simulink model "Ackerman_simulation"  (R2024b)
settings: Solver=VariableStepAuto  StartTime=0.0  StopTime=inf  RelTol=1e-3
values from neighbouring files (symbols this model uses):
  psi_o = 0    [PursuitWaypoints.m]
  Ts = 200    [PursuitWaypoints.m]    (also in retardo.m = 0.01)
  X_end = refPose(end,1)    [PursuitWaypoints.m]
  X_o = refPose(1,1)    [PursuitWaypoints.m]
  xRef = interp1(1:length(xRef), xRef, puntos_finos, 'spline')'    [PursuitWaypoints.m]
  Y_end = -refPose(end,2)    [PursuitWaypoints.m]
  Y_o = -refPose(1,2)    [PursuitWaypoints.m]
  yRef = interp1(1:length(yRef), yRef, puntos_finos, 'spline')'    [PursuitWaypoints.m]
undefined symbols (not defined in the file or in its folder): DiscIntNeverNeededParam
libraries: simulink x6, robotalgslib x2, robotmobilelib x1
settings Model: Creator=johan  LastModifiedBy=johan
settings OptimizationCC: DefaultParameterBehavior=Inlined  GainParamInheritBuiltInType=on  UseFloatMulNetSlope=on  InlineInvariantSignals=on  EfficientFloat2IntCast=on
settings RTWCC: RTWVerbose=off  BuildConfiguration=Faster Runs
settings GRTTargetCC: MatFileLogging=off

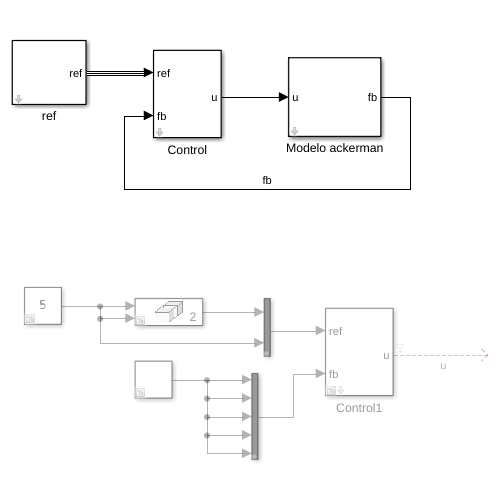
[thumbnail: Simulink's stored preview of the top-level diagram]
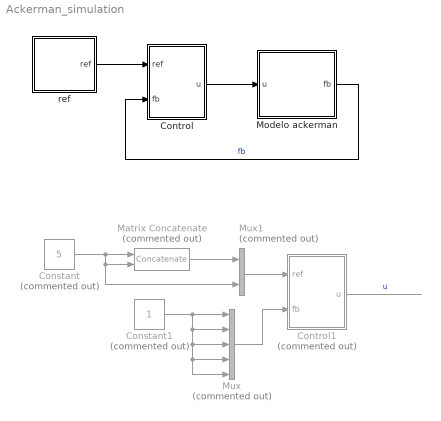
== system Ackerman_simulation ==
  Constant : Constant  Commented=on  Value=5
  Constant1 : Constant  Commented=on
  Control : Subsystem  mask{Kp=5, Ki=1.25, psi_kp=5, psi_ki=1, Error_pos=2, Simulation_end=1000}
      mask prompts: Kp "Proportional (Kp):"; Ki "Integral (Ki):"; psi_kp "Proportional (Kp):"; psi_ki "Integral (Ki):"; Error_pos "Error pos"; Simulation_end "Simulation end:"
      mask DialogControl ParameterGroupVar Prompt: Control parameters
      mask DialogControl Container3 Prompt: Speed gains
      mask DialogControl Container4 Prompt: Direction gains
      mask DialogControl Container6 Prompt: Simulation config
  Control1 : Subsystem  Commented=on  mask{Ki=1.25, Kp=5, Error_pos=1, Simulation_end=1000}
      mask prompts: Ki "Integral (Ki):"; Kp "Proportional (Kp):"; Error_pos "Error pos"; Simulation_end "Simulation end:"
      mask DialogControl ParameterGroupVar Prompt: Control gains
      mask DialogControl Container6 Prompt: Simulation config
  Matrix Concatenate : Concatenate  Commented=on  Mode=Multidimensional array  ConcatenateDimension=2
  Modelo ackerman : Subsystem  mask{angular_limit=pi/4, speed_limit=10, wheel_base=1.5, m=5, Crr=0.015, alpha=30}
      mask prompts: angular_limit "Limite angular:"; speed_limit "Limite velocidad:"; wheel_base "Distancia ruedas (L):"; m "Masa (m):"; Crr "Resistencia rodadura (Crr):"; alpha "Angulo terreno (alpha):"
      mask DialogControl ParameterGroupVar Prompt: Model limits
      mask DialogControl Container2 Prompt: Model parameters
  Mux : Mux  Commented=on  Inputs=5
  Mux1 : Mux  Commented=on  Inputs=2
  ref : Subsystem  mask{spd_ref=2}
      mask prompts: spd_ref "Speed ref:"
      mask DialogControl DescGroupVar Prompt: Description
      mask DialogControl DescTextVar Prompt: Mask to introduce waypoints. Expected same size for x and y.
      mask DialogControl ParameterGroupVar Prompt: References
  wires:
  Modelo ackerman/1(fb) -> Control/2(fb)  "fb"
  ref/1(ref) -> Control/1(ref)
  Control/1(u) -> Modelo ackerman/1(u)
  Control1/1(u) -> ?  "u"
  Matrix Concatenate/1 -> Mux1/1
  Constant/1 -> Mux1/2, Matrix Concatenate/2, Matrix Concatenate/1
  Constant1/1 -> Mux/5, Mux/4, Mux/3, Mux/2, Mux/1
  Mux/1 -> Control1/2(fb)
  Mux1/1 -> Control1/1(ref)

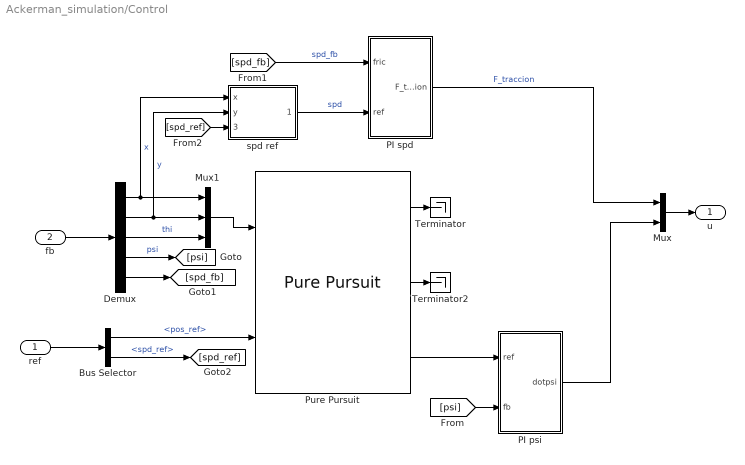
== system Ackerman_simulation/Control ==
  ref : Inport
  fb : Inport  Port=2
  Bus Selector : BusSelector  OutputSignals=pos_ref,spd_ref
  Demux : Demux  Outputs=5
  Mux : Mux  Inputs=2
  Mux1 : Mux  Inputs=3
  PI psi : Subsystem
  PI spd : Subsystem
  Pure Pursuit : robotalgslib/Pure Pursuit  DesiredLinearVelocityPort=off  DesiredLinearVelocity=1  MaxAngularVelocity=1.0  LookaheadDistancePort=off  LookaheadDistance=ld  TargetDirPort=on  SimulateUsing=Code generation
      settings: LibrarySourceBlock=robotmobilelib/Pure Pursuit
  Terminator : Terminator
  Terminator2 : Terminator
  "spd ref " : Subsystem  mask{Error_pos=Error_pos, Simulation_end=Simulation_end}
      mask prompts: Error_pos "Error pos:"; Simulation_end "Simulation time end:"
  u : Outport
  wires:
  fb/1 -> Demux/1
  Demux/1 -> "spd ref "/1(x), Mux1/1  "x"
  Demux/2 -> "spd ref "/2(y), Mux1/2  "y"
  Demux/3 -> Mux1/3  "thi"
  Mux1/1 -> Pure Pursuit/1
  ref/1 -> Bus Selector/1
  Pure Pursuit/1 -> Terminator/1
  Pure Pursuit/3 -> PI psi/1(ref)
  Demux/4 -> [psi]  "psi"
  Pure Pursuit/2 -> Terminator2/1
  [psi] -> PI psi/2(fb)
  PI spd/1(F_traccion) -> Mux/1  "F_traccion"
  Mux/1 -> u/1
  "spd ref "/1(spd ref) -> PI spd/2(ref)  "spd"
  Demux/5 -> [spd_fb]
  [spd_fb] -> PI spd/1(fric)  "spd_fb"
  Bus Selector/1 -> Pure Pursuit/2  "<pos_ref>"
  Bus Selector/2 -> [spd_ref]  "<spd_ref>"
  [spd_ref] -> "spd ref "/3(spd_ref)
  PI psi/1(dotpsi) -> Mux/2

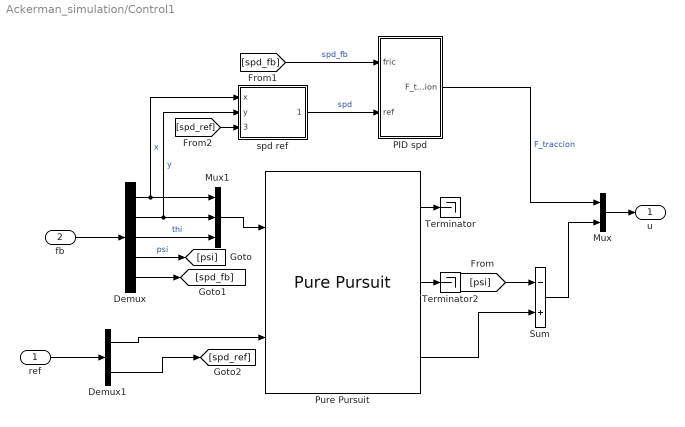
== system Ackerman_simulation/Control1 ==
  ref : Inport
  fb : Inport  Port=2
  Demux : Demux  Outputs=5
  Demux1 : Demux  Outputs=2
  Mux : Mux  Inputs=2
  Mux1 : Mux  Inputs=3
  PID spd : Subsystem
  Pure Pursuit : robotalgslib/Pure Pursuit  DesiredLinearVelocityPort=off  DesiredLinearVelocity=1  MaxAngularVelocity=1.0  LookaheadDistancePort=off  LookaheadDistance=ld  TargetDirPort=on  SimulateUsing=Code generation
      settings: LibrarySourceBlock=robotmobilelib/Pure Pursuit
  Sum : Sum  Inputs=-+
  Terminator : Terminator
  Terminator2 : Terminator
  "spd ref " : Subsystem  mask{Error_pos=Error_pos, Simulation_end=Simulation_end}
      mask prompts: Error_pos "Error pos:"; Simulation_end "Simulation time end:"
  u : Outport
  wires:
  [spd_ref] -> "spd ref "/3(spd_ref)
  Demux1/2 -> [spd_ref]
  [spd_fb] -> PID spd/1(fric)  "spd_fb"
  Demux/5 -> [spd_fb]
  "spd ref "/1(spd ref) -> PID spd/2(ref)  "spd"
  Mux/1 -> u/1
  PID spd/1(F_traccion) -> Mux/1  "F_traccion"
  [psi] -> Sum/1
  Sum/1 -> Mux/2
  Pure Pursuit/2 -> Terminator2/1
  Demux/4 -> [psi]  "psi"
  Pure Pursuit/3 -> Sum/2
  Pure Pursuit/1 -> Terminator/1
  ref/1 -> Demux1/1
  Mux1/1 -> Pure Pursuit/1
  Demux/3 -> Mux1/3  "thi"
  Demux/2 -> Mux1/2, "spd ref "/2(y)  "y"
  Demux/1 -> Mux1/1, "spd ref "/1(x)  "x"
  fb/1 -> Demux/1
  Demux1/1 -> Pure Pursuit/2

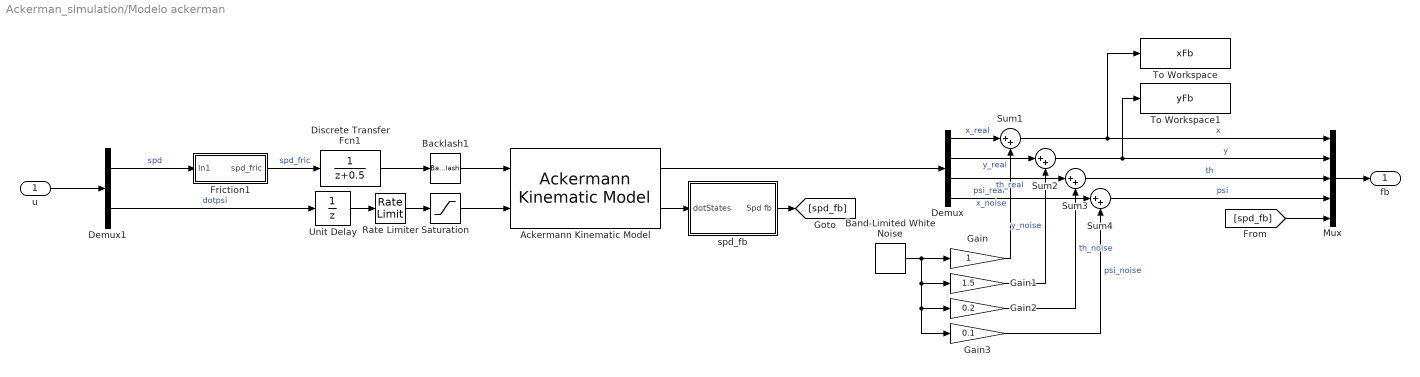
== system Ackerman_simulation/Modelo ackerman ==
  u : Inport
  Ackermann Kinematic Model : robotmobilelib/Ackermann Kinematic Model  WheelBase=wheel_base  VehicleSpeedRange=[-speed_limit speed_limit]  MaxSteeringAngle=1  InitialState=[X_o; Y_o; 0; psi_o]  SimulateUsing=Code generation
  Backlash1 : Backlash  BacklashWidth=0.05
  Band-Limited White Noise : simulink/Sources/Band-Limited White Noise  Cov=[0.001]  Ts=0.1  seed=[23341]
  Demux : Demux
  Demux1 : Demux  Outputs=2
  Discrete Transfer Fcn1 : DiscreteTransferFcn
  Friction1 : Subsystem  mask{m=m, alpha=alpha, Crr=Crr}
      mask prompts: m "Masa (m):"; alpha "Angulo terreno (alpha):"; Crr "Resistencia rodadura (Crr):"
  Gain : Gain
  Gain1 : Gain  Gain=1.5
  Gain2 : Gain  Gain=0.2
  Gain3 : Gain  Gain=0.1
  Mux : Mux  Inputs=5
  Rate Limiter : RateLimiter  RisingSlewLimit=2  FallingSlewLimit=-2  SampleTimeMode=inherited
  Saturation : Saturate  UpperLimit=angular_limit  LowerLimit=-angular_limit
  Sum{1..4} (4 alike) : Sum  Inputs=|++
  To Workspace : ToWorkspace  VariableName=xFb  SaveFormat=Timeseries  SampleTime=-1
  To Workspace1 : ToWorkspace  VariableName=yFb  SaveFormat=Timeseries  SampleTime=-1
  Unit Delay : UnitDelay  SampleTime=-1  HasFrameUpgradeWarning=on
  spd_fb : Subsystem
  fb : Outport
  wires:
  Sum1/1 -> To Workspace/1, Mux/1  "x"
  Sum2/1 -> To Workspace1/1, Mux/2  "y"
  Mux/1 -> fb/1
  Sum4/1 -> Mux/4  "psi"
  Ackermann Kinematic Model/2 -> spd_fb/1(dotStates)
  Sum3/1 -> Mux/3  "th"
  Ackermann Kinematic Model/1 -> Demux/1
  Demux/1 -> Sum1/1  "x_real"
  Demux/2 -> Sum2/1  "y_real"
  Demux/4 -> Sum4/1  "psi_real"
  Demux/3 -> Sum3/1  "th_real"
  Gain/1 -> Sum1/2  "x_noise"
  Gain1/1 -> Sum2/2  "y_noise"
  Gain2/1 -> Sum3/2  "th_noise"
  Gain3/1 -> Sum4/2  "psi_noise"
  Band-Limited White Noise/1 -> Gain2/1, Gain3/1, Gain1/1, Gain/1
  Unit Delay/1 -> Rate Limiter/1
  Rate Limiter/1 -> Saturation/1
  u/1 -> Demux1/1
  Saturation/1 -> Ackermann Kinematic Model/2
  Demux1/1 -> Friction1/1(In1)  "spd"
  Demux1/2 -> Unit Delay/1  "dotpsi"
  Friction1/1(spd_fric) -> Discrete Transfer Fcn1/1  "spd_fric"
  [spd_fb] -> Mux/5
  spd_fb/1(Spd fb) -> [spd_fb]
  Backlash1/1 -> Ackermann Kinematic Model/1
  Discrete Transfer Fcn1/1 -> Backlash1/1

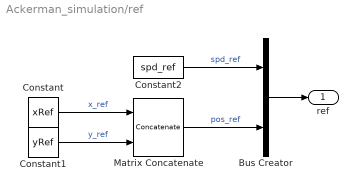
== system Ackerman_simulation/ref ==
  Bus Creator : BusCreator  Inputs=2
  Constant : Constant  Value=xRef  SampleTime=Ts
  Constant1 : Constant  Value=yRef  SampleTime=Ts
  Constant2 : Constant  Value=spd_ref  SampleTime=Ts
  Matrix Concatenate : Concatenate  Mode=Multidimensional array  ConcatenateDimension=2
  ref : Outport
  wires:
  Constant1/1 -> Matrix Concatenate/2  "y_ref"
  Constant/1 -> Matrix Concatenate/1  "x_ref"
  Matrix Concatenate/1 -> Bus Creator/2  "pos_ref"
  Constant2/1 -> Bus Creator/1  "spd_ref"
  Bus Creator/1 -> ref/1

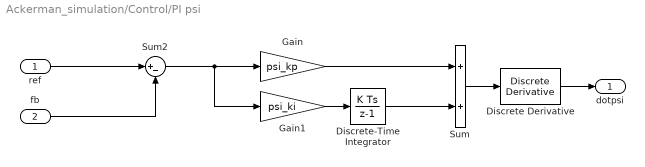
== system Ackerman_simulation/Control/PI psi ==
  ref : Inport
  fb : Inport  Port=2
  Discrete Derivative : simulink/Discrete/Discrete Derivative  gainval=1.0  ICPrevScaledInput=0.0  OutMin=[]  OutMax=[]  OutDataType=fixdt(1, 16)  OutScaling=2^-10  DoSatur=off
  Discrete-Time Integrator : DiscreteIntegrator  SampleTime=-1  ICPrevOutput=DiscIntNeverNeededParam  ICPrevScaledInput=DiscIntNeverNeededParam
  Gain : Gain  Gain=psi_kp
  Gain1 : Gain  Gain=psi_ki
  Sum : Sum
  Sum2 : Sum  Inputs=|+-
  dotpsi : Outport
  wires:
  Gain1/1 -> Discrete-Time Integrator/1
  ref/1 -> Sum2/1
  Gain/1 -> Sum/1
  Discrete-Time Integrator/1 -> Sum/2
  Sum/1 -> Discrete Derivative/1
  Sum2/1 -> Gain1/1, Gain/1
  fb/1 -> Sum2/2
  Discrete Derivative/1 -> dotpsi/1

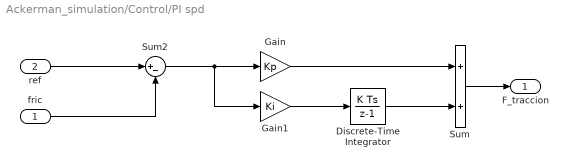
== system Ackerman_simulation/Control/PI spd ==
  fric : Inport
  ref : Inport  Port=2
  Discrete-Time Integrator : DiscreteIntegrator  SampleTime=-1  ICPrevOutput=DiscIntNeverNeededParam  ICPrevScaledInput=DiscIntNeverNeededParam
  Gain : Gain  Gain=Kp
  Gain1 : Gain  Gain=Ki
  Sum : Sum
  Sum2 : Sum  Inputs=|+-
  F_traccion : Outport
  wires:
  Gain1/1 -> Discrete-Time Integrator/1
  ref/1 -> Sum2/1
  Gain/1 -> Sum/1
  Discrete-Time Integrator/1 -> Sum/2
  Sum/1 -> F_traccion/1
  Sum2/1 -> Gain1/1, Gain/1
  fric/1 -> Sum2/2

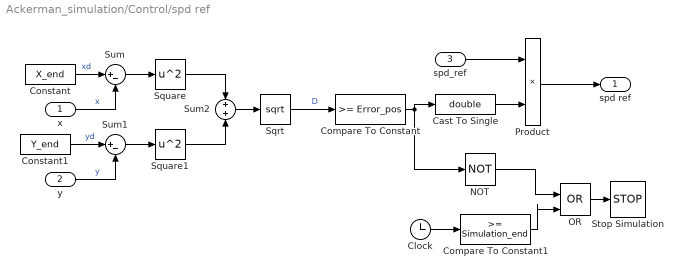
== system Ackerman_simulation/Control/spd ref  ==
  x : Inport
  y : Inport  Port=2
  spd_ref : Inport  Port=3
  Cast To Single : DataTypeConversion  OutDataTypeStr=double  SaturateOnIntegerOverflow=off  RndMeth=Floor
  Clock : Clock
  Compare To Constant : simulink/Logic and Bit Operations/Compare To Constant  relop=>=  const=Error_pos  OutDataTypeStr=uint8
  Compare To Constant1 : simulink/Logic and Bit Operations/Compare To Constant  relop=>=  const=Simulation_end  OutDataTypeStr=boolean
  Constant : Constant  Value=X_end
  Constant1 : Constant  Value=Y_end
  NOT : Logic  Operator=NOT  IconShape=distinctive  AllPortsSameDT=off  OutDataTypeStr=boolean
  OR : Logic  Operator=OR  IconShape=distinctive  AllPortsSameDT=off  OutDataTypeStr=boolean
  Product : Product
  Sqrt : Sqrt
  Square : Math  Operator=square
  Square1 : Math  Operator=square
  Stop Simulation : Stop
  Sum : Sum  Inputs=|+-
  Sum1 : Sum  Inputs=|+-
  Sum2 : Sum
  spd ref : Outport
  wires:
  Constant/1 -> Sum/1  "xd"
  x/1 -> Sum/2  "x"
  Constant1/1 -> Sum1/1  "yd"
  y/1 -> Sum1/2  "y"
  Sum/1 -> Square/1
  Sum1/1 -> Square1/1
  Square1/1 -> Sum2/2
  Square/1 -> Sum2/1
  Sum2/1 -> Sqrt/1
  Sqrt/1 -> Compare To Constant/1  "D"
  Product/1 -> spd ref/1
  Compare To Constant/1 -> NOT/1, Cast To Single/1
  Cast To Single/1 -> Product/2
  NOT/1 -> OR/1
  Clock/1 -> Compare To Constant1/1
  Compare To Constant1/1 -> OR/2
  OR/1 -> Stop Simulation/1
  spd_ref/1 -> Product/1

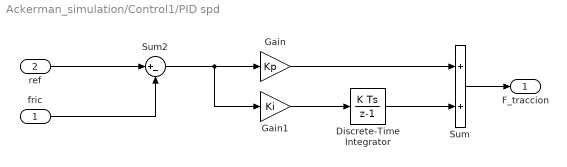
== system Ackerman_simulation/Control1/PID spd ==
  fric : Inport
  ref : Inport  Port=2
  Discrete-Time Integrator : DiscreteIntegrator  SampleTime=-1  ICPrevOutput=DiscIntNeverNeededParam  ICPrevScaledInput=DiscIntNeverNeededParam
  Gain : Gain  Gain=Kp
  Gain1 : Gain  Gain=Ki
  Sum : Sum
  Sum2 : Sum  Inputs=|+-
  F_traccion : Outport
  wires:
  fric/1 -> Sum2/2
  Sum2/1 -> Gain/1, Gain1/1
  Sum/1 -> F_traccion/1
  Discrete-Time Integrator/1 -> Sum/2
  Gain/1 -> Sum/1
  ref/1 -> Sum2/1
  Gain1/1 -> Discrete-Time Integrator/1

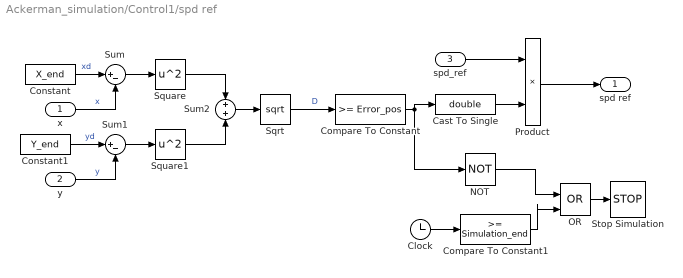
== system Ackerman_simulation/Control1/spd ref  ==
  x : Inport
  y : Inport  Port=2
  spd_ref : Inport  Port=3
  Cast To Single : DataTypeConversion  OutDataTypeStr=double  SaturateOnIntegerOverflow=off  RndMeth=Floor
  Clock : Clock
  Compare To Constant : simulink/Logic and Bit Operations/Compare To Constant  relop=>=  const=Error_pos  OutDataTypeStr=uint8
  Compare To Constant1 : simulink/Logic and Bit Operations/Compare To Constant  relop=>=  const=Simulation_end  OutDataTypeStr=boolean
  Constant : Constant  Value=X_end
  Constant1 : Constant  Value=Y_end
  NOT : Logic  Operator=NOT  IconShape=distinctive  AllPortsSameDT=off  OutDataTypeStr=boolean
  OR : Logic  Operator=OR  IconShape=distinctive  AllPortsSameDT=off  OutDataTypeStr=boolean
  Product : Product
  Sqrt : Sqrt
  Square : Math  Operator=square
  Square1 : Math  Operator=square
  Stop Simulation : Stop
  Sum : Sum  Inputs=|+-
  Sum1 : Sum  Inputs=|+-
  Sum2 : Sum
  spd ref : Outport
  wires:
  spd_ref/1 -> Product/1
  OR/1 -> Stop Simulation/1
  Compare To Constant1/1 -> OR/2
  Clock/1 -> Compare To Constant1/1
  NOT/1 -> OR/1
  Cast To Single/1 -> Product/2
  Compare To Constant/1 -> Cast To Single/1, NOT/1
  Product/1 -> spd ref/1
  Sqrt/1 -> Compare To Constant/1  "D"
  Sum2/1 -> Sqrt/1
  Square/1 -> Sum2/1
  Square1/1 -> Sum2/2
  Sum1/1 -> Square1/1
  Sum/1 -> Square/1
  y/1 -> Sum1/2  "y"
  Constant1/1 -> Sum1/1  "yd"
  x/1 -> Sum/2  "x"
  Constant/1 -> Sum/1  "xd"

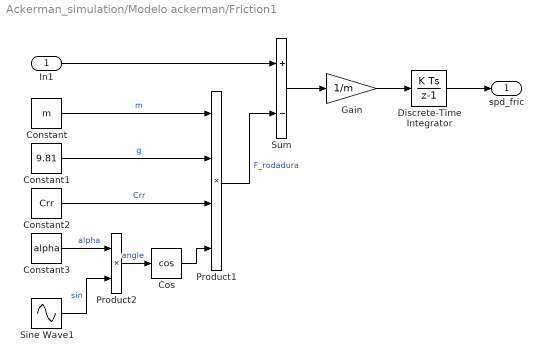
== system Ackerman_simulation/Modelo ackerman/Friction1 ==
  In1 : Inport
  Constant : Constant  Value=m
  Constant1 : Constant  Value=9.81
  Constant2 : Constant  Value=Crr
  Constant3 : Constant  Value=alpha
  Cos : Trigonometry  Operator=cos
  Discrete-Time Integrator : DiscreteIntegrator  SampleTime=-1  ICPrevOutput=DiscIntNeverNeededParam  ICPrevScaledInput=DiscIntNeverNeededParam
  Gain : Gain  Gain=1/m
  Product1 : Product  Inputs=4
  Product2 : Product
  Sine Wave1 : Sin  SampleTime=0
  Sum : Sum  Inputs=+-
  spd_fric : Outport
  wires:
  Sum/1 -> Gain/1
  In1/1 -> Sum/1
  Discrete-Time Integrator/1 -> spd_fric/1
  Gain/1 -> Discrete-Time Integrator/1
  Product1/1 -> Sum/2  "F_rodadura"
  Constant2/1 -> Product1/3  "Crr"
  Cos/1 -> Product1/4
  Constant3/1 -> Product2/1  "alpha"
  Constant1/1 -> Product1/2  "g"
  Constant/1 -> Product1/1  "m"
  Product2/1 -> Cos/1  "angle"
  Sine Wave1/1 -> Product2/2  "sin"

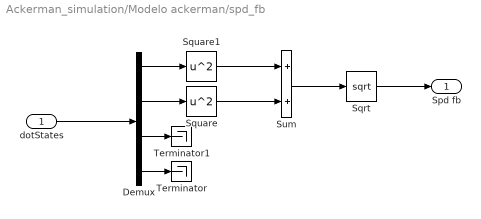
== system Ackerman_simulation/Modelo ackerman/spd_fb ==
  dotStates : Inport
  Demux : Demux
  Sqrt : Sqrt
  Square : Math  Operator=square
  Square1 : Math  Operator=square
  Sum : Sum
  Terminator : Terminator
  Terminator1 : Terminator
  Spd fb : Outport
  wires:
  dotStates/1 -> Demux/1
  Demux/4 -> Terminator/1
  Demux/3 -> Terminator1/1
  Demux/1 -> Square1/1
  Demux/2 -> Square/1
  Square1/1 -> Sum/1
  Square/1 -> Sum/2
  Sum/1 -> Sqrt/1
  Sqrt/1 -> Spd fb/1
